simulink model "AM_DSB_TC_RXsolucio"  (R2024b)
settings: Solver=VariableStepAuto  StartTime=0.0  StopTime=inf  RelTol=1e-3
libraries: dspsnks4 x1, dspmlti4 x1, sdrrlib x1
settings Model: Creator=javier.alonsov  LastModifiedBy=javier.alonsov

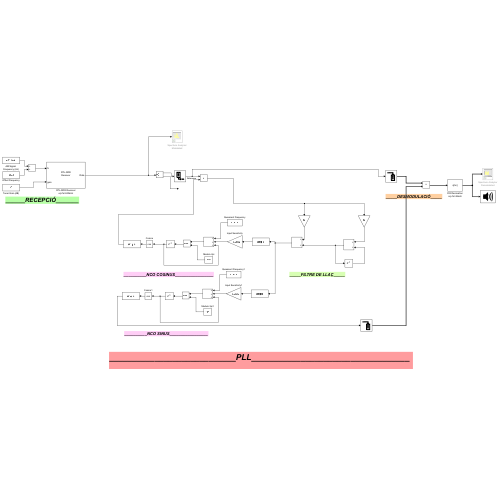
[thumbnail: Simulink's stored preview of the top-level diagram]
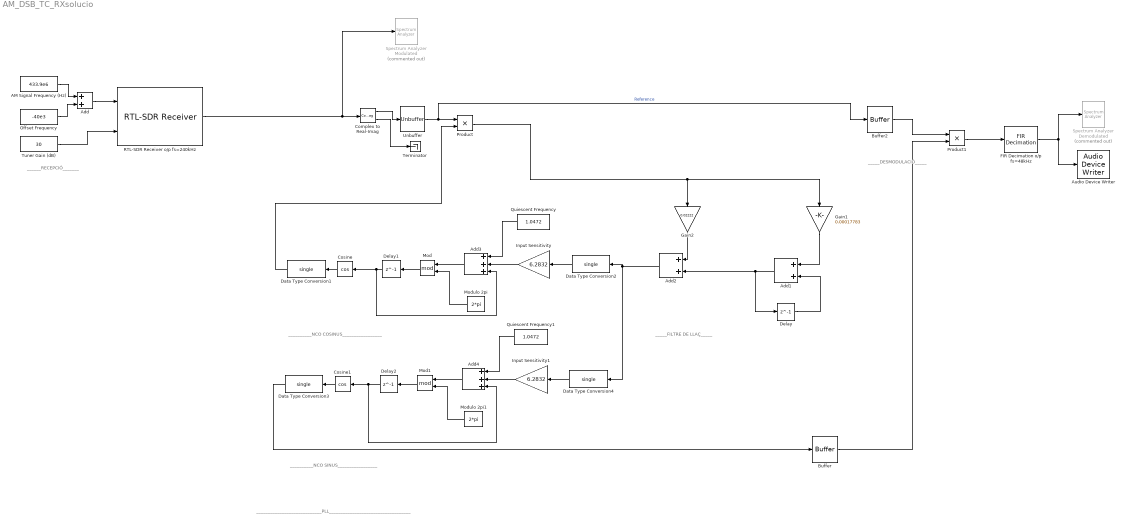
== system AM_DSB_TC_RXsolucio ==
  note: _____DESMODULACIÓ_____
  note: _____FILTRE DE LLAÇ_____
  note: __________NCO COSINUS_________________
  note: __________NCO SINUS_________________
  note: ____________________________PLL___________________________________
  note: ______RECEPCIÓ_______
  AM Signal Frequency (Hz) : Constant  Value=433.9e6
  Add : Sum
  Add1 : Sum
  Add2 : Sum  OutDataTypeStr=single  AccumDataTypeStr=single
  Add3 : Sum  Inputs=+++
  Add4 : Sum  Inputs=+++
  Audio Device Writer : dspsnks4/Audio Device Writer  Driver=DirectSound  Device=Default  InheritSampleRate=on  SampleRate=44100  BitDepth=16-bit integer  BufferSize=4096  NumBuffers=10  DefaultOutputChannelMapping=on  OutputChannelMapping=1:2  OutputNumUnderrunSamples=off  DriverIdx=1  DeviceWarnFlag=''
  Buffer : Buffer  N=4096
  Buffer2 : Buffer  N=4096
  Complex to Real-Imag : ComplexToRealImag
  Cosine : Trigonometry  Operator=cos  OutputSignalType=real
  Cosine1 : Trigonometry  Operator=cos  OutputSignalType=real
  Data Type Conversion{1..4} (4 alike) : DataTypeConversion  OutDataTypeStr=single  SaturateOnIntegerOverflow=off  RndMeth=Floor
  Delay : Delay  DelayLength=1  InitialCondition=0.00
  Delay1 : Delay  DelayLength=1  InitialCondition=0
  Delay2 : Delay  DelayLength=1  InitialCondition=pi/2
  FIR Decimation o/p fs=48kHz : dspmlti4/FIR Decimation  FilterSource=Dialog parameters  h=firpm(200, [0 15e3 20e3 (240e3/2)]/(240e3/2), [1 1 0 0], [1 1], 20)  D=5  filtStruct=Direct form  FilterObject=Hm_firdecim  InputProcessing=Columns as channels (frame based)  framing=Allow multirate processing  AllowArbitraryInputLength=off  inputOffset=0  outputBufInitCond=0  roundingMode=Floor  overflowMode=off  firstCoeffDataTypeStr=Inherit: Same word length as input  firstCoeffMin=[]  firstCoeffMax=[]  firstCoeffLastDataTypeStr=Inherit: Same word length as input  outputDataTypeStr=Inherit: Same as accumulator  outputMin=[]  outputMax=[]  outputLastDataTypeStr=Inherit: Same as accumulator
  Gain1 : Gain  Gain=0.00017783  OutDataTypeStr=single
  Gain2 : Gain  Gain=0.02222  ParamDataTypeStr=single
  Input Sensitivity : Gain  Gain=6.2832
  Input Sensitivity1 : Gain  Gain=6.2832
  Mod : Math  Operator=mod
  Mod1 : Math  Operator=mod
  Modulo 2pi : Constant  Value=2*pi  SampleTime=1/240e3
  Modulo 2pi1 : Constant  Value=2*pi  SampleTime=1/240e3
  Offset Frequency : Constant  Value=-40e3
  Product : Product
  Product1 : Product
  Quiescent Frequency : Constant  Value=1.0472  SampleTime=1/240e3
  Quiescent Frequency1 : Constant  Value=1.0472  SampleTime=1/240e3
  RTL-SDR Receiver o/p fs=240kHz : sdrrlib/RTL-SDR Receiver  IPAddress=0  CenterFrequencySource=Input port  CenterFrequency=433.9e6-100e3  GainSource=Input port  Gain=40  ADCRate=240e3  FrequencyCorrection=0  LostSamplesOutputPort=off  LatencyOutputPort=off  OutputDataType=single  FrameLength=4096  EnableBurstMode=off  NumFramesInBurst=20  sobjType=sdrr.internal.SDRRTLReceiverSL  dataUDPPort=-1  ctrlUDPPort=-1  subDeviceList=nosubdev  sdrBlockType=SDRBlockTypeSLT.SDRRxBlock  requester=UNUSED_BY_SFCN  sdrExecutionMode=SDRExecutionModeSLT.ExecModeHW  BypassUserLogic=off  DecimatorSelect=DDC decimator  SourceSelect=RF data  SineAmplitude=16000  EnableInternalClock=off  BypassIQBalance=off  IFBandwidth=40e6  ADCRateSource=Dialog  IntermediateFrequency=0  DecimationFactorSource=Dialog  DecimationFactor=512  RFFrequencyIsTunable=logical(1)  SampleTime=(4096)/(240e3)  IFBandwidthSource=Dialog  SineFrequency=30000  BypassDCBlockingFilter=off  IntermediateFrequencySource=Dialog  IQBalanceCoefficients=64  SkipAllHardwareResetAndInitialization=off  EnableIQCalibrationTable=on  CacheIQCalibrationTable=off  EnableOffsetTuning=off  EnableRTLAGC=off  EnableTestMode=off  EnableTunerAGC=off  FrequencyCorrectionSource=Dialog  NumMLBuffers=128  NumUSBBuffers=16  RTLCrystalFrequency=28800000  TunerCrystalFrequency=28800000
  Spectrum Analyzer Demodulated : SpectrumAnalyzer  Commented=on  WindowPosition=[1070.000000,603.000000,778.000000,224.000000,]  ScopeFrameLocation=window  Method=Welch  SampleRate=48000  AxesScaling=Manual  Span=240000  StartFrequency=-120000  StopFrequency=120000  AveragingMethod=Running  YLimits=[-180.94415229593105,48.14480110113395]  AllowFFTLengthLessThanSamplesPerUpdate=on  DefaultConfigurationName=spbscopes.SpectrumAnalyzerBlockCfg  IsFrequencyInputMode=0  FrequencyVectorPort=0  FrequencyVectorFromPort=0  FrequencyInputRBWPort=0  FrequencyInputRBWFromPort=0
  Spectrum Analyzer Modulated : SpectrumAnalyzer  Commented=on  WindowPosition=[1070.000000,261.000000,777.000000,407.000000,]  Visible=on  ScopeFrameLocation=window  Method=Welch  SampleRate=240000  AxesScaling=Manual  Span=240000  StartFrequency=-120000  StopFrequency=120000  AveragingMethod=Running  YLimits=[-146.72067730693476,43.804014640077718]  AllowFFTLengthLessThanSamplesPerUpdate=on  DefaultConfigurationName=spbscopes.SpectrumAnalyzerBlockCfg  IsFrequencyInputMode=0  FrequencyVectorPort=0  FrequencyVectorFromPort=0  FrequencyInputRBWPort=0  FrequencyInputRBWFromPort=0
  Terminator : Terminator
  Tuner Gain (dB) : Constant  Value=30
  Unbuffer : Unbuffer
  wires:
  Offset Frequency/1 -> Add/2
  AM Signal Frequency (Hz)/1 -> Add/1
  Tuner Gain (dB)/1 -> RTL-SDR Receiver o/p fs=240kHz/2
  Add/1 -> RTL-SDR Receiver o/p fs=240kHz/1
  FIR Decimation o/p fs=48kHz/1 -> Audio Device Writer/1, Spectrum Analyzer Demodulated/1
  RTL-SDR Receiver o/p fs=240kHz/1 -> Complex to Real-Imag/1, Spectrum Analyzer Modulated/1
  Complex to Real-Imag/2 -> Terminator/1
  Complex to Real-Imag/1 -> Unbuffer/1
  Unbuffer/1 -> Buffer2/1, Product/1  "Reference"
  Gain2/1 -> Add2/1
  Product/1 -> Gain2/1, Gain1/1
  Gain1/1 -> Add1/1
  Delay/1 -> Add1/2
  Add1/1 -> Delay/1, Add2/2
  Data Type Conversion2/1 -> Input Sensitivity/1
  Input Sensitivity/1 -> Add3/2
  Quiescent Frequency/1 -> Add3/1
  Modulo 2pi/1 -> Mod/2
  Add3/1 -> Mod/1
  Mod/1 -> Delay1/1
  Delay1/1 -> Cosine/1, Add3/3
  Cosine/1 -> Data Type Conversion1/1
  Modulo 2pi1/1 -> Mod1/2
  Quiescent Frequency1/1 -> Add4/1
  Cosine1/1 -> Data Type Conversion3/1
  Add4/1 -> Mod1/1
  Data Type Conversion4/1 -> Input Sensitivity1/1
  Delay2/1 -> Cosine1/1, Add4/3
  Add2/1 -> Data Type Conversion2/1, Data Type Conversion4/1
  Input Sensitivity1/1 -> Add4/2
  Mod1/1 -> Delay2/1
  Data Type Conversion1/1 -> Product/2
  Product1/1 -> FIR Decimation o/p fs=48kHz/1
  Buffer2/1 -> Product1/1
  Buffer/1 -> Product1/2
  Data Type Conversion3/1 -> Buffer/1
